simulink model "SERIALMASTERUPDATED"  (R2022b)
settings: Solver=FixedStepAuto  StartTime=0.0  StopTime=10.0  FixedStep=1e-3  RelTol=1e-3  EnableMultiTasking=on
undefined symbols (not defined in the file): D0, D1, D10, D11, D12, D13, D2, D3, D4, D5, D6, D7, D8, D9, PTA0, PTA1, PTA2, PTB23, PTB9, PTC16, PTC17, PTC2, PTC3, PTC4, PTD0, PTD1, PTD2, PTD3
libraries: frdmk64flib x18, etargetslib x12
settings Model: ExtModeTrigDuration=5  Creator=Riley  LastModifiedBy=Tiren
settings OptimizationCC: EnhancedBackFolding=on  PassReuseOutputArgsAs=Individual arguments  ZeroExternalMemoryAtStartup=off  ZeroInternalMemoryAtStartup=off  MaxStackSize=64  OptimizeBlockOrder=speed  DifferentSizesBufferReuse=on  OptimizationCustomize=off  EfficientTunableParamExpr=on
settings DebuggingCC: ParameterTunabilityLossMsg=error  UnconnectedInputMsg=warning  UnconnectedOutputMsg=warning  UnconnectedLineMsg=warning
settings HardwareCC: ProdBitPerPointer=32  ProdBitPerSizeT=32  ProdBitPerPtrDiffT=32  ProdLargestAtomicInteger=Long  ProdLargestAtomicFloat=Double  ProdWordSize=32  ProdHWDeviceType=ARM Compatible->ARM Cortex
settings ModelReferenceCC: EnableRefExpFcnMdlSchedulingChecks=on
settings SFSimCC: MATLABDynamicMemAlloc=off
settings RTWCC: Description=Embedded Coder  SystemTargetFile=ert.tlc  HardwareBoard=NXP FRDM-K64F  TLCOptions="-aInlineSetEventsForThisBaseRateFcn=TLC_FALSE -aSuppressMultiTaskScheduler=TLC_FALSE  -aRateBasedStepFcn=0"  TemplateMakefile=ert_default_tmf  Toolchain=GNU Tools for ARM Embedded Processors  DLArmComputeVersion=19.05
settings CodeAppCC: ForceParamTrailComments=on  IgnoreCustomStorageClasses=off  OperatorAnnotations=on  SimulinkDataObjDesc=on  SFDataObjDesc=on  InsertBlockDesc=on
settings ERTTargetCC: ExtModeTransport=4  ExtModeMexFile=sendToCommService

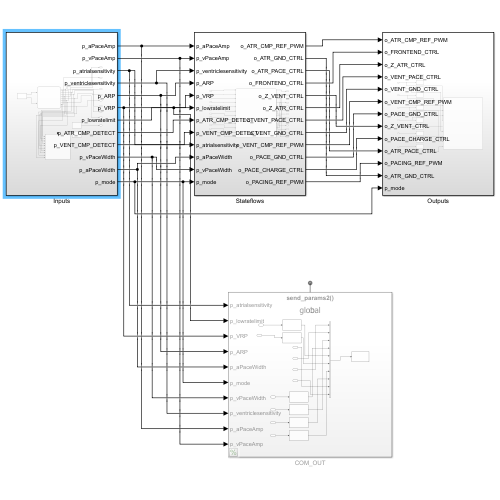
[thumbnail: Simulink's stored preview of the top-level diagram]
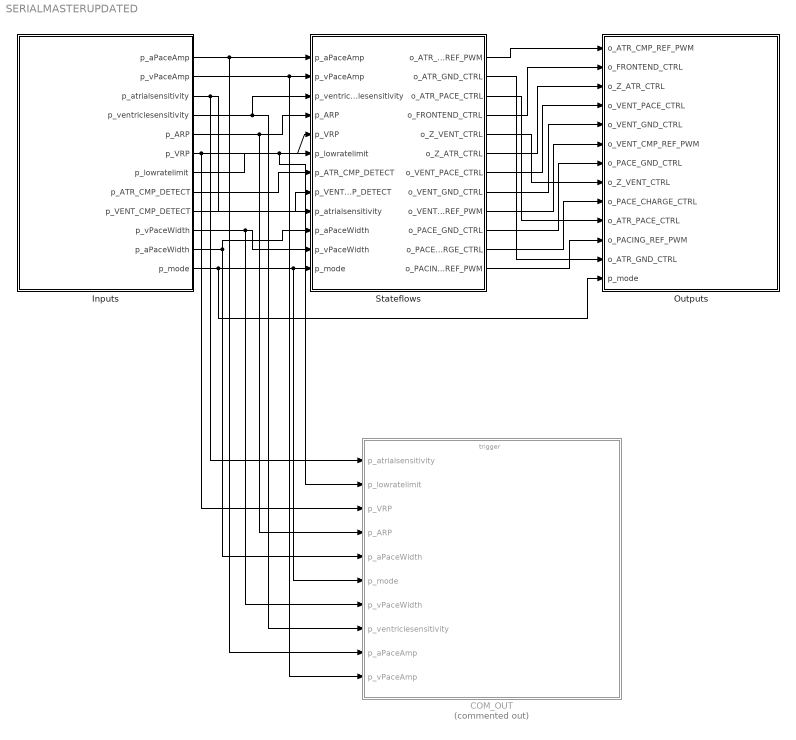
== system SERIALMASTERUPDATED ==
  COM_OUT : Subsystem  Commented=on  TreatAsAtomicUnit=on
  Inputs : Subsystem
  Outputs : Subsystem
  Stateflows : Subsystem
  wires:
  Inputs/1(p_aPaceAmp) -> COM_OUT/9(p_aPaceAmp), Stateflows/1(p_aPaceAmp)
  Inputs/2(p_vPaceAmp) -> COM_OUT/10(p_vPaceAmp), Stateflows/2(p_vPaceAmp)
  Inputs/3(p_atrialsensitivity) -> COM_OUT/1(p_atrialsensitivity), Stateflows/9(p_atrialsensitivity)
  Inputs/4(p_ventriclesensitivity) -> COM_OUT/8(p_ventriclesensitivity), Stateflows/3(p_ventriclesensitivity)
  Inputs/5(p_ARP) -> COM_OUT/4(p_ARP), Stateflows/4(p_ARP)
  Inputs/6(p_VRP) -> COM_OUT/3(p_VRP), Stateflows/5(p_VRP)
  Inputs/7(p_lowratelimit) -> COM_OUT/2(p_lowratelimit), Stateflows/6(p_lowratelimit)
  Inputs/8(p_ATR_CMP_DETECT) -> Stateflows/7(p_ATR_CMP_DETECT)
  Inputs/9(p_VENT_CMP_DETECT) -> Stateflows/8(p_VENT_CMP_DETECT)
  Inputs/10(p_vPaceWidth) -> COM_OUT/7(p_vPaceWidth), Stateflows/11(p_vPaceWidth)
  Inputs/11(p_aPaceWidth) -> COM_OUT/5(p_aPaceWidth), Stateflows/10(p_aPaceWidth)
  Inputs/12(p_mode) -> Outputs/13(p_mode), COM_OUT/6(p_mode), Stateflows/12(p_mode)
  Stateflows/1(o_ATR_CMP_REF_PWM) -> Outputs/1(o_ATR_CMP_REF_PWM)
  Stateflows/2(o_ATR_GND_CTRL) -> Outputs/12(o_ATR_GND_CTRL)
  Stateflows/3(o_ATR_PACE_CTRL) -> Outputs/10(o_ATR_PACE_CTRL)
  Stateflows/4(o_FRONTEND_CTRL) -> Outputs/2(o_FRONTEND_CTRL)
  Stateflows/5(o_Z_VENT_CTRL) -> Outputs/8(o_Z_VENT_CTRL)
  Stateflows/6(o_Z_ATR_CTRL) -> Outputs/3(o_Z_ATR_CTRL)
  Stateflows/7(o_VENT_PACE_CTRL) -> Outputs/4(o_VENT_PACE_CTRL)
  Stateflows/8(o_VENT_GND_CTRL) -> Outputs/5(o_VENT_GND_CTRL)
  Stateflows/9(o_VENT_CMP_REF_PWM) -> Outputs/6(o_VENT_CMP_REF_PWM)
  Stateflows/10(o_PACE_GND_CTRL) -> Outputs/7(o_PACE_GND_CTRL)
  Stateflows/11(o_PACE_CHARGE_CTRL) -> Outputs/9(o_PACE_CHARGE_CTRL)
  Stateflows/12(o_PACING_REF_PWM) -> Outputs/11(o_PACING_REF_PWM)

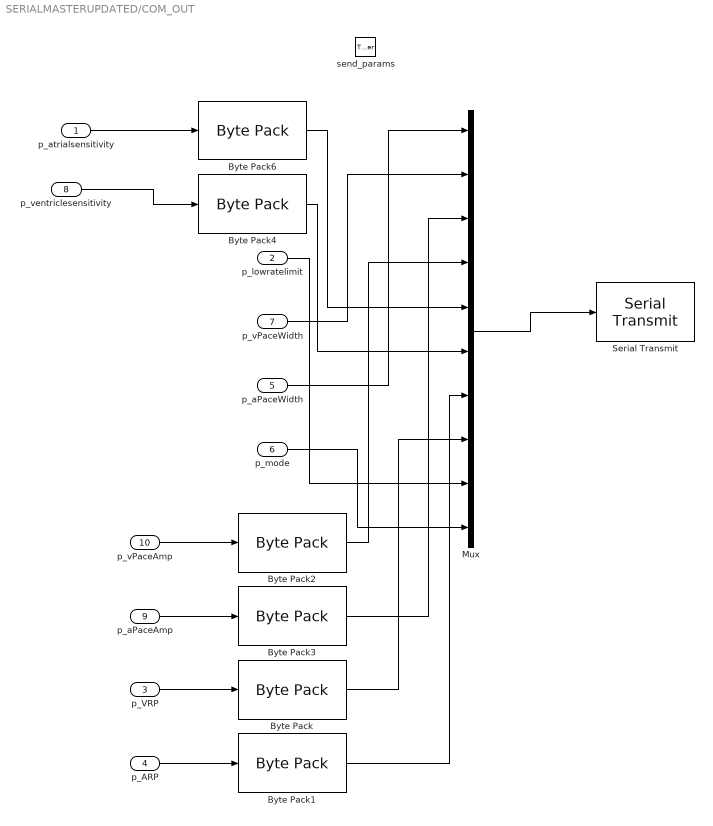
== system SERIALMASTERUPDATED/COM_OUT ==
  p_atrialsensitivity : Inport  OutDataTypeStr=single
  p_lowratelimit : Inport  Port=2  OutDataTypeStr=uint8
  p_VRP : Inport  Port=3  OutDataTypeStr=uint16
  p_ARP : Inport  Port=4  OutDataTypeStr=uint16
  p_aPaceWidth : Inport  Port=5  OutDataTypeStr=uint8
  p_mode : Inport  Port=6  OutDataTypeStr=uint8
  p_vPaceWidth : Inport  Port=7  OutDataTypeStr=uint8
  p_ventriclesensitivity : Inport  Port=8  OutDataTypeStr=single
  p_aPaceAmp : Inport  Port=9  OutDataTypeStr=single
  p_vPaceAmp : Inport  Port=10  OutDataTypeStr=single
  send_params : TriggerPort  TriggerType=function-call  IsSimulinkFunction=on  FunctionName=send_params2  VariantControl=(inherit)
  Byte Pack : etargetslib/Byte Pack  datatypes={'uint16'}  byteAlign=1
  Byte Pack1 : etargetslib/Byte Pack  datatypes={'uint16'}  byteAlign=1
  Byte Pack{2..4,6} (4 alike) : etargetslib/Byte Pack  datatypes={'single'}  byteAlign=1
  Mux : Mux  Inputs=10
  Serial Transmit : frdmk64flib/Serial Transmit  SCIModule=0  Baudrate=uint32(9600)  Parity=None  StopBits=1  HardwareFlowControl=None  ByteOrder=LittleEndian  BlockingMode=on  OutputStatus=off
  wires:
  Mux/1 -> Serial Transmit/1
  p_VRP/1 -> Byte Pack/1
  p_ARP/1 -> Byte Pack1/1
  p_vPaceAmp/1 -> Byte Pack2/1
  p_aPaceAmp/1 -> Byte Pack3/1
  p_atrialsensitivity/1 -> Byte Pack6/1
  p_ventriclesensitivity/1 -> Byte Pack4/1
  p_aPaceWidth/1 -> Mux/1
  p_vPaceWidth/1 -> Mux/2
  Byte Pack3/1 -> Mux/3
  Byte Pack2/1 -> Mux/4
  Byte Pack6/1 -> Mux/5
  Byte Pack4/1 -> Mux/6
  Byte Pack1/1 -> Mux/7
  Byte Pack/1 -> Mux/8
  p_lowratelimit/1 -> Mux/9
  p_mode/1 -> Mux/10

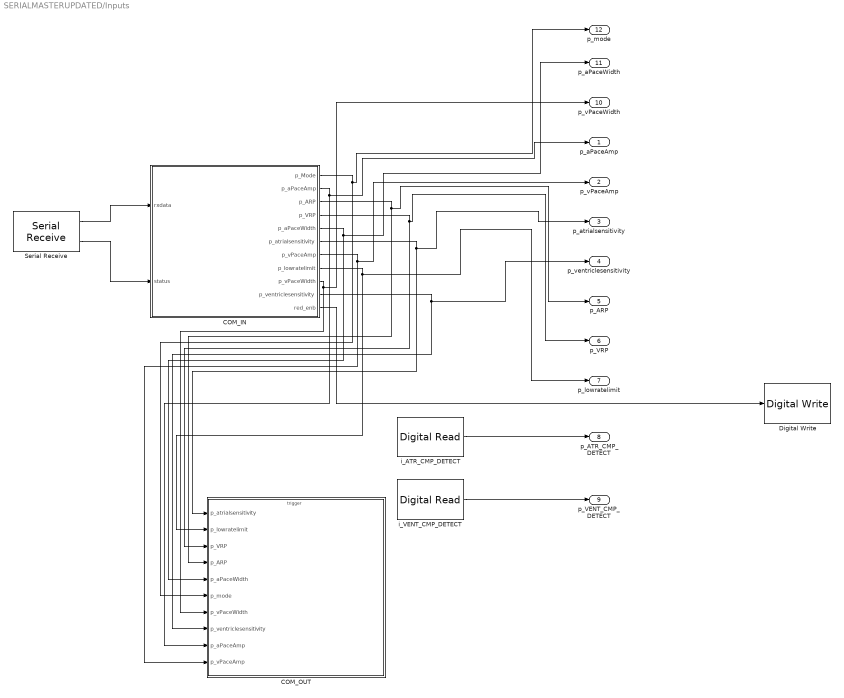
== system SERIALMASTERUPDATED/Inputs ==
  COM_IN : Stateflow chart  TreatAsAtomicUnit=on
  COM_OUT : Subsystem  TreatAsAtomicUnit=on
  Digital Write : frdmk64flib/Digital Write  Whichpin=RED_LED
  Serial Receive : frdmk64flib/Serial Receive  SCIModule=0  Baudrate=uint32(9600)  Parity=None  StopBits=1  HardwareFlowControl=None  ByteOrder=LittleEndian  DataType=uint8  DataLength=26  BlockingMode=off  OutputStatus=on  SampleTime=0.1
  i_ATR_CMP_DETECT : frdmk64flib/Digital Read  Whichpin=PTC16 (D0)  SampleTime=-1
  i_VENT_CMP_DETECT : frdmk64flib/Digital Read  Whichpin=PTC17 (D1)  SampleTime=-1
  p_aPaceAmp : Outport  OutDataTypeStr=single  Unit=mV
  p_vPaceAmp : Outport  Port=2  OutDataTypeStr=single  Unit=mV
  p_atrialsensitivity : Outport  Port=3  OutDataTypeStr=single  Unit=mV
  p_ventriclesensitivity : Outport  Port=4  OutDataTypeStr=single  Unit=mV
  p_ARP : Outport  Port=5  OutDataTypeStr=uint16  Unit=msec
  p_VRP : Outport  Port=6  OutDataTypeStr=uint16  Unit=msec
  p_lowratelimit : Outport  Port=7  OutDataTypeStr=uint8  Unit=msec
  p_ATR_CMP_DETECT : Outport  Port=8  OutDataTypeStr=boolean
  p_VENT_CMP_DETECT : Outport  Port=9  OutDataTypeStr=boolean
  p_vPaceWidth : Outport  Port=10  OutDataTypeStr=uint8  Unit=msec
  p_aPaceWidth : Outport  Port=11  OutDataTypeStr=uint8  Unit=msec
  p_mode : Outport  Port=12  OutDataTypeStr=uint8
  wires:
  i_ATR_CMP_DETECT/1 -> p_ATR_CMP_DETECT/1
  i_VENT_CMP_DETECT/1 -> p_VENT_CMP_DETECT/1
  Serial Receive/1 -> COM_IN/1(rxdata)
  Serial Receive/2 -> COM_IN/2(status)
  COM_IN/1(p_Mode) -> COM_OUT/6(p_mode), p_mode/1
  COM_IN/3(p_ARP) -> COM_OUT/4(p_ARP), p_ARP/1
  COM_IN/4(p_VRP) -> COM_OUT/3(p_VRP), p_VRP/1
  COM_IN/2(p_aPaceAmp) -> COM_OUT/9(p_aPaceAmp), p_aPaceAmp/1
  COM_IN/5(p_aPaceWidth) -> COM_OUT/5(p_aPaceWidth), p_aPaceWidth/1
  COM_IN/6(p_atrialsensitivity) -> COM_OUT/1(p_atrialsensitivity), p_atrialsensitivity/1
  COM_IN/8(p_lowratelimit) -> COM_OUT/2(p_lowratelimit), p_lowratelimit/1
  COM_IN/10(p_ventriclesensitivity) -> COM_OUT/8(p_ventriclesensitivity), p_ventriclesensitivity/1
  COM_IN/9(p_vPaceWidth) -> COM_OUT/7(p_vPaceWidth), p_vPaceWidth/1
  COM_IN/7(p_vPaceAmp) -> p_vPaceAmp/1, COM_OUT/10(p_vPaceAmp)
  COM_IN/11(red_enb) -> Digital Write/1

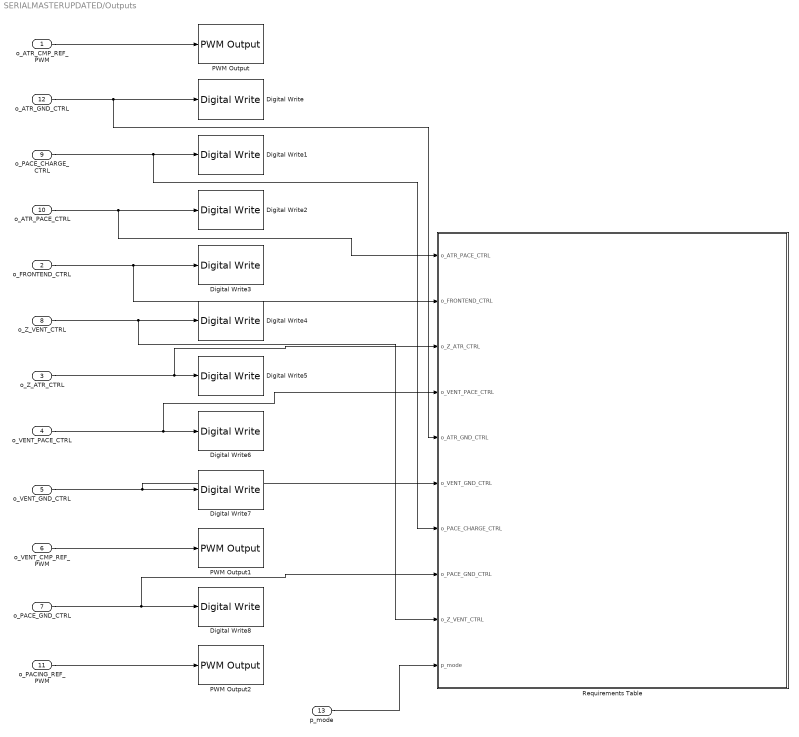
== system SERIALMASTERUPDATED/Outputs ==
  o_ATR_CMP_REF_PWM : Inport  OutDataTypeStr=single
  o_FRONTEND_CTRL : Inport  Port=2  OutDataTypeStr=boolean
  o_Z_ATR_CTRL : Inport  Port=3  OutDataTypeStr=boolean
  o_VENT_PACE_CTRL : Inport  Port=4  OutDataTypeStr=boolean
  o_VENT_GND_CTRL : Inport  Port=5  OutDataTypeStr=boolean
  o_VENT_CMP_REF_PWM : Inport  Port=6  OutDataTypeStr=single
  o_PACE_GND_CTRL : Inport  Port=7  OutDataTypeStr=boolean
  o_Z_VENT_CTRL : Inport  Port=8  OutDataTypeStr=boolean
  o_PACE_CHARGE_CTRL : Inport  Port=9  OutDataTypeStr=boolean
  o_ATR_PACE_CTRL : Inport  Port=10  OutDataTypeStr=boolean
  o_PACING_REF_PWM : Inport  Port=11  OutDataTypeStr=single
  o_ATR_GND_CTRL : Inport  Port=12  OutDataTypeStr=boolean
  p_mode : Inport  Port=13  OutDataTypeStr=uint8
  Digital Write : frdmk64flib/Digital Write  Whichpin=PTD2 (D11)
  Digital Write1 : frdmk64flib/Digital Write  Whichpin=PTB9 (D2)
  Digital Write2 : frdmk64flib/Digital Write  Whichpin=PTA0 (D8)
  Digital Write3 : frdmk64flib/Digital Write  Whichpin=PTD1 (D13)
  Digital Write4 : frdmk64flib/Digital Write  Whichpin=PTC3 (D7)
  Digital Write5 : frdmk64flib/Digital Write  Whichpin=PTB23 (D4)
  Digital Write6 : frdmk64flib/Digital Write  Whichpin=PTC4 (D9)
  Digital Write7 : frdmk64flib/Digital Write  Whichpin=PTD3 (D12)
  Digital Write8 : frdmk64flib/Digital Write  Whichpin=PTD0 (D10)
  PWM Output : frdmk64flib/PWM Output  Whichpin=PTC2 (D6)  InitialFrequency=2000  InitialDutyCycle=0
  PWM Output1 : frdmk64flib/PWM Output  Whichpin=PTA1 (D3)  InitialFrequency=2000  InitialDutyCycle=0
  PWM Output2 : frdmk64flib/PWM Output  Whichpin=PTA2 (D5)  InitialFrequency=2000  InitialDutyCycle=0
  Requirements Table : Requirements Table  TreatAsAtomicUnit=on
  wires:
  o_ATR_CMP_REF_PWM/1 -> PWM Output/1
  o_ATR_GND_CTRL/1 -> Requirements Table/5(o_ATR_GND_CTRL), Digital Write/1
  o_PACE_CHARGE_CTRL/1 -> Requirements Table/7(o_PACE_CHARGE_CTRL), Digital Write1/1
  o_ATR_PACE_CTRL/1 -> Requirements Table/1(o_ATR_PACE_CTRL), Digital Write2/1
  o_FRONTEND_CTRL/1 -> Requirements Table/2(o_FRONTEND_CTRL), Digital Write3/1
  o_Z_VENT_CTRL/1 -> Requirements Table/9(o_Z_VENT_CTRL), Digital Write4/1
  o_Z_ATR_CTRL/1 -> Requirements Table/3(o_Z_ATR_CTRL), Digital Write5/1
  o_VENT_PACE_CTRL/1 -> Requirements Table/4(o_VENT_PACE_CTRL), Digital Write6/1
  o_VENT_GND_CTRL/1 -> Requirements Table/6(o_VENT_GND_CTRL), Digital Write7/1
  o_VENT_CMP_REF_PWM/1 -> PWM Output1/1
  o_PACE_GND_CTRL/1 -> Requirements Table/8(o_PACE_GND_CTRL), Digital Write8/1
  o_PACING_REF_PWM/1 -> PWM Output2/1
  p_mode/1 -> Requirements Table/10(p_mode)

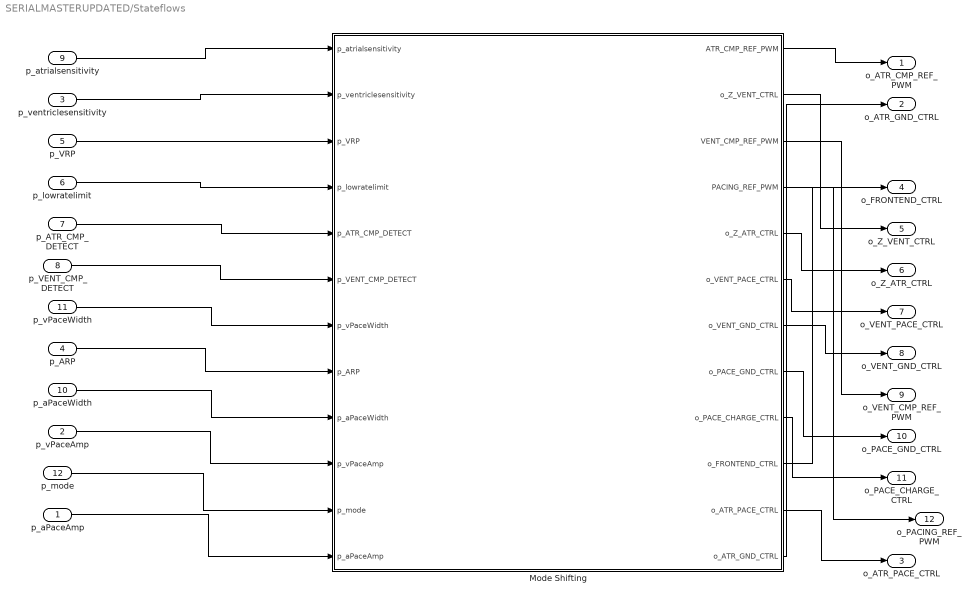
== system SERIALMASTERUPDATED/Stateflows ==
  p_aPaceAmp : Inport  OutDataTypeStr=single
  p_vPaceAmp : Inport  Port=2  OutDataTypeStr=single
  p_ventriclesensitivity : Inport  Port=3  OutDataTypeStr=single
  p_ARP : Inport  Port=4  OutDataTypeStr=uint16
  p_VRP : Inport  Port=5  OutDataTypeStr=uint16
  p_lowratelimit : Inport  Port=6  OutDataTypeStr=uint8
  p_ATR_CMP_DETECT : Inport  Port=7  OutDataTypeStr=boolean
  p_VENT_CMP_DETECT : Inport  Port=8  OutDataTypeStr=boolean
  p_atrialsensitivity : Inport  Port=9  OutDataTypeStr=single
  p_aPaceWidth : Inport  Port=10  OutDataTypeStr=uint8
  p_vPaceWidth : Inport  Port=11  OutDataTypeStr=uint8
  p_mode : Inport  Port=12  OutDataTypeStr=uint8
  Mode Shifting : Stateflow chart  TreatAsAtomicUnit=on
  o_ATR_CMP_REF_PWM : Outport  OutDataTypeStr=single
  o_ATR_GND_CTRL : Outport  Port=2  OutDataTypeStr=boolean
  o_ATR_PACE_CTRL : Outport  Port=3  OutDataTypeStr=boolean
  o_FRONTEND_CTRL : Outport  Port=4  OutDataTypeStr=boolean
  o_Z_VENT_CTRL : Outport  Port=5  OutDataTypeStr=boolean
  o_Z_ATR_CTRL : Outport  Port=6  OutDataTypeStr=boolean
  o_VENT_PACE_CTRL : Outport  Port=7  OutDataTypeStr=boolean
  o_VENT_GND_CTRL : Outport  Port=8  OutDataTypeStr=boolean
  o_VENT_CMP_REF_PWM : Outport  Port=9  OutDataTypeStr=single
  o_PACE_GND_CTRL : Outport  Port=10  OutDataTypeStr=boolean
  o_PACE_CHARGE_CTRL : Outport  Port=11  OutDataTypeStr=boolean
  o_PACING_REF_PWM : Outport  Port=12  OutDataTypeStr=single
  wires:
  p_aPaceAmp/1 -> Mode Shifting/12(p_aPaceAmp)
  p_vPaceAmp/1 -> Mode Shifting/10(p_vPaceAmp)
  p_atrialsensitivity/1 -> Mode Shifting/1(p_atrialsensitivity)
  p_ventriclesensitivity/1 -> Mode Shifting/2(p_ventriclesensitivity)
  p_ARP/1 -> Mode Shifting/8(p_ARP)
  p_VRP/1 -> Mode Shifting/3(p_VRP)
  p_lowratelimit/1 -> Mode Shifting/4(p_lowratelimit)
  p_ATR_CMP_DETECT/1 -> Mode Shifting/5(p_ATR_CMP_DETECT)
  p_VENT_CMP_DETECT/1 -> Mode Shifting/6(p_VENT_CMP_DETECT)
  p_vPaceWidth/1 -> Mode Shifting/7(p_vPaceWidth)
  p_aPaceWidth/1 -> Mode Shifting/9(p_aPaceWidth)
  p_mode/1 -> Mode Shifting/11(p_mode)
  Mode Shifting/1(ATR_CMP_REF_PWM) -> o_ATR_CMP_REF_PWM/1
  Mode Shifting/2(o_Z_VENT_CTRL) -> o_Z_VENT_CTRL/1
  Mode Shifting/3(VENT_CMP_REF_PWM) -> o_VENT_CMP_REF_PWM/1
  Mode Shifting/4(PACING_REF_PWM) -> o_PACING_REF_PWM/1
  Mode Shifting/5(o_Z_ATR_CTRL) -> o_Z_ATR_CTRL/1
  Mode Shifting/6(o_VENT_PACE_CTRL) -> o_VENT_PACE_CTRL/1
  Mode Shifting/7(o_VENT_GND_CTRL) -> o_VENT_GND_CTRL/1
  Mode Shifting/8(o_PACE_GND_CTRL) -> o_PACE_GND_CTRL/1
  Mode Shifting/9(o_PACE_CHARGE_CTRL) -> o_PACE_CHARGE_CTRL/1
  Mode Shifting/10(o_FRONTEND_CTRL) -> o_FRONTEND_CTRL/1
  Mode Shifting/11(o_ATR_PACE_CTRL) -> o_ATR_PACE_CTRL/1
  Mode Shifting/12(o_ATR_GND_CTRL) -> o_ATR_GND_CTRL/1

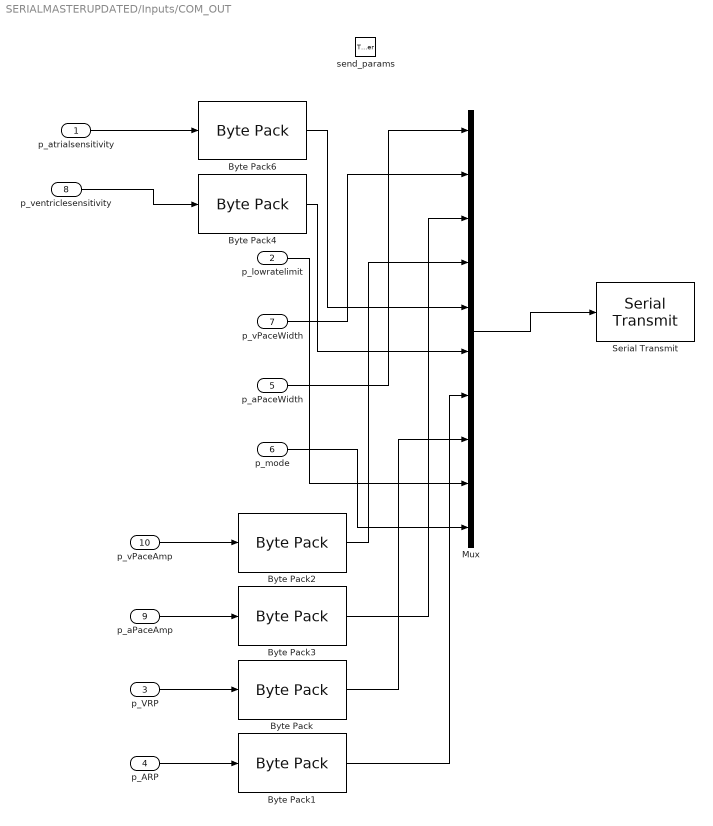
== system SERIALMASTERUPDATED/Inputs/COM_OUT ==
  p_atrialsensitivity : Inport  OutDataTypeStr=single
  p_lowratelimit : Inport  Port=2  OutDataTypeStr=uint8
  p_VRP : Inport  Port=3  OutDataTypeStr=uint16
  p_ARP : Inport  Port=4  OutDataTypeStr=uint16
  p_aPaceWidth : Inport  Port=5  OutDataTypeStr=uint8
  p_mode : Inport  Port=6  OutDataTypeStr=uint8
  p_vPaceWidth : Inport  Port=7  OutDataTypeStr=uint8
  p_ventriclesensitivity : Inport  Port=8  OutDataTypeStr=single
  p_aPaceAmp : Inport  Port=9  OutDataTypeStr=single
  p_vPaceAmp : Inport  Port=10  OutDataTypeStr=single
  send_params : TriggerPort  TriggerType=function-call  IsSimulinkFunction=on  FunctionName=send_params2  VariantControl=(inherit)
  Byte Pack : etargetslib/Byte Pack  datatypes={'uint16'}  byteAlign=1
  Byte Pack1 : etargetslib/Byte Pack  datatypes={'uint16'}  byteAlign=1
  Byte Pack{2..4,6} (4 alike) : etargetslib/Byte Pack  datatypes={'single'}  byteAlign=1
  Mux : Mux  Inputs=10
  Serial Transmit : frdmk64flib/Serial Transmit  SCIModule=0  Baudrate=uint32(9600)  Parity=None  StopBits=1  HardwareFlowControl=None  ByteOrder=LittleEndian  BlockingMode=on  OutputStatus=off
  wires:
  Mux/1 -> Serial Transmit/1
  p_VRP/1 -> Byte Pack/1
  p_ARP/1 -> Byte Pack1/1
  p_vPaceAmp/1 -> Byte Pack2/1
  p_aPaceAmp/1 -> Byte Pack3/1
  p_atrialsensitivity/1 -> Byte Pack6/1
  p_ventriclesensitivity/1 -> Byte Pack4/1
  p_aPaceWidth/1 -> Mux/1
  p_vPaceWidth/1 -> Mux/2
  Byte Pack3/1 -> Mux/3
  Byte Pack2/1 -> Mux/4
  Byte Pack6/1 -> Mux/5
  Byte Pack4/1 -> Mux/6
  Byte Pack1/1 -> Mux/7
  Byte Pack/1 -> Mux/8
  p_lowratelimit/1 -> Mux/9
  p_mode/1 -> Mux/10

== stateflow chart SERIALMASTERUPDATED/Inputs/COM_IN ==
  state SET_PARAMETERS
    entry:
    p_aPaceWidth = rxdata(3);
    p_vPaceWidth = rxdata(4);
    p_aPaceAmp = typecast(rxdata(5:8),'single');
    p_vPaceAmp = typecast(rxdata(9:12),'single');
    p_atrialsensitivity = typecast(rxdata(13:16),'single');
    p_ventriclesensitivity = typecast(rxdata(17:20),'single');
    p_ARP = typecast(rxdata(21:22),'uint16');
    p_VRP =typecast(rxdata(23:24),'uint16');
    p_lowratelimit = rxdata(25);
    p_Mode = rxdata(26);
    %red_enb = 1;
  state INITIAL
    %Set the initial values of parameters
    entry:
    p_aPaceWidth = 5;
    p_vPaceWidth = 1;
    p_aPaceAmp = 1;
    p_vPaceAmp = 1;
    p_atrialsensitivity = 1;
    p_ventriclesensitivity = 1;
    p_ARP = 1;
    p_VRP = 1;
    p_lowratelimit = 1;
    p_Mode =1;
    red_enb = 0;
  state STANDBY
    %wait for COM
  state ECHO_PARAMETERS
    entry:
    send_params2();
    red_enb = 1;
  SET_PARAMETERS -> STANDBY
  (default) -> INITIAL
  (junction 12) -> SET_PARAMETERS [order 2] : [rxdata(2)==55]
  (junction 9) -> STANDBY [order 2]
  INITIAL -> STANDBY
  STANDBY -> (junction 9) : [status == 0]
  (junction 9) -> (junction 12) [order 1] : [rxdata(1) == hex2dec('16')]
  (junction 12) -> ECHO_PARAMETERS [order 1] : [rxdata(2)==hex2dec('22')]
  ECHO_PARAMETERS -> STANDBY
  data: rxdata input uint8; status input uint8; p_Mode output uint8; p_aPaceAmp output single; p_ARP output uint16; p_VRP output uint16; p_aPaceWidth output uint8; p_atrialsensitivity output single; p_vPaceAmp output single; p_lowratelimit output uint8; p_vPaceWidth output uint8; p_ventriclesensitivity output single; red_enb output

== stateflow chart SERIALMASTERUPDATED/Stateflows/Mode Shifting ==
  state AOOPACING
    entry:
    %AV pacing
    o_PACE_CHARGE_CTRL= false;
    o_PACE_GND_CTRL = true;
    o_ATR_PACE_CTRL = true;
    o_ATR_GND_CTRL = false;
    o_VENT_GND_CTRL = false;
    o_VENT_PACE_CTRL =  false;
  state VOOPACING
    entry:
    %AV pacing
    o_PACE_CHARGE_CTRL= false;
    o_PACE_GND_CTRL = true;
    o_ATR_PACE_CTRL = false;
    o_ATR_GND_CTRL = false;
    o_VENT_GND_CTRL = false;
    o_VENT_PACE_CTRL =  true;
  state AAIPACINGHEART
    entry:
    %AV pacing
    o_PACE_CHARGE_CTRL= false;
    o_PACE_GND_CTRL = true;
    o_ATR_PACE_CTRL = true;
    o_ATR_GND_CTRL = false;
    o_VENT_GND_CTRL = false;
    o_VENT_PACE_CTRL =  false;
    %SENSING OFF
    o_FRONTEND_CTRL = false;
  state VVIPACINGHEART
    entry:
    %AV pacing
    o_PACE_CHARGE_CTRL= false;
    o_PACE_GND_CTRL = true;
    o_ATR_PACE_CTRL = false;
    o_ATR_GND_CTRL = false;
    o_VENT_GND_CTRL = false;
    o_VENT_PACE_CTRL =  true;
    %SENSING OFF
    o_FRONTEND_CTRL = false;
  state AAIDETECTION
    entry:
    %SENSING ON
    o_FRONTEND_CTRL = true;
  state VVIDETECTION
    entry:
    %SENSING ON
    o_FRONTEND_CTRL = true;
  state AOOCHARGINGDISCHARGING
    entry:
    %To charge C22
    o_ATR_PACE_CTRL = false;
    o_PACE_CHARGE_CTRL = true;
    %To discharge blocking capacitor
    entry:
    o_PACE_GND_CTRL = true;
    o_VENT_PACE_CTRL = false;
    o_ATR_PACE_CTRL = false;
    o_ATR_GND_CTRL = true;
  state VOOCHARGINGDISCHARGING
    entry:
    %To charge C22
    o_VENT_PACE_CTRL = false;
    o_PACE_CHARGE_CTRL = true;
    o_ATR_PACE_CTRL = false;
    %To discharge blocking capacitor
    entry:
    o_PACE_GND_CTRL = true;
    o_VENT_PACE_CTRL = false;
    o_ATR_PACE_CTRL = false;
    o_VENT_GND_CTRL = true;
  state AAICHARGINGDISCHARGING
    entry:
    %To charge C22
    o_ATR_PACE_CTRL = false;
    o_PACE_CHARGE_CTRL = true;
    %To discharge blocking capacitor
    entry:
    o_PACE_GND_CTRL = true;
    o_VENT_PACE_CTRL = false;
    o_ATR_PACE_CTRL = false;
    o_ATR_GND_CTRL = true;
  state VVICHARGINGDISCHARGING
    entry:
    %To charge C22
    o_VENT_PACE_CTRL = false;
    o_PACE_CHARGE_CTRL = true;
    o_ATR_PACE_CTRL = false;
    %To discharge blocking capacitor
    entry:
    o_PACE_GND_CTRL = true;
    o_VENT_PACE_CTRL = false;
    o_ATR_PACE_CTRL = false;
    o_VENT_GND_CTRL = true;
  state DEFAULTSTATE
    o_Z_ATR_CTRL = false;
    o_Z_VENT_CTRL = false;
    o_VENT_PACE_CTRL = false;
    o_ATR_PACE_CTRL = false;
    VPACING_REF_PWM = (p_vPaceAmp/5000)*100;
    APACING_REF_PWM = (p_aPaceAmp/5000)*100;
    o_FRONTEND_CTRL = false;
    ATR_CMP_REF_PWM = (p_atrialsensitivity/5000)*100;
    VENT_CMP_REF_PWM = (p_ventriclesensitivity/5000)*100;
    o_PACE_CHARGE_CTRL = false;
    o_ATR_GND_CTRL = false;
    o_VENT_GND_CTRL = false;
    o_PACE_GND_CTRL = false;
  VVIPACINGHEART -> VVICHARGINGDISCHARGING
  AAIPACINGHEART -> AAICHARGINGDISCHARGING : after(p_aPaceWidth,msec)
  AOOCHARGINGDISCHARGING -> AOOPACING : after(p_lowratelimit - p_aPaceWidth,msec)
  AOOPACING -> AOOCHARGINGDISCHARGING : after(p_aPaceWidth,msec)
  VOOCHARGINGDISCHARGING -> VOOPACING : after(p_lowratelimit - p_vPaceWidth,msec)
  VOOPACING -> VOOCHARGINGDISCHARGING : after(p_vPaceWidth,msec)
  AAIDETECTION -> AAIPACINGHEART [order 2] : after(p_lowratelimit-p_aPaceWidth-uint8(p_ARP),msec)
  VVIDETECTION -> VVIPACINGHEART [order 2] : after(p_lowratelimit-p_vPaceWidth-uint8(p_VRP),msec)
  VVIDETECTION -> VVICHARGINGDISCHARGING [order 1] : [p_VENT_CMP_DETECT == true]
  AAIDETECTION -> AAICHARGINGDISCHARGING [order 1] : [p_ATR_CMP_DETECT == true]
  AAICHARGINGDISCHARGING -> AAIDETECTION : after(p_ARP,msec)
  VVICHARGINGDISCHARGING -> VVIDETECTION : after(p_VRP,msec)
  DEFAULTSTATE -> AOOCHARGINGDISCHARGING [order 2] : [p_mode == 1]{PACING_REF_PWM = APACING_REF_PWM}
  DEFAULTSTATE -> VOOCHARGINGDISCHARGING [order 1] : [p_mode == 2 ]{PACING_REF_PWM = APACING_REF_PWM}
  DEFAULTSTATE -> AAICHARGINGDISCHARGING [order 3] : [p_mode == 3]{PACING_REF_PWM = VPACING_REF_PWM}
  DEFAULTSTATE -> VVICHARGINGDISCHARGING [order 4] : [p_mode == 4]{PACING_REF_PWM = VPACING_REF_PWM}
  (default) -> DEFAULTSTATE
  data: p_atrialsensitivity input single; p_ventriclesensitivity input single; p_VRP input uint16; p_lowratelimit input uint8; p_ATR_CMP_DETECT input boolean; p_VENT_CMP_DETECT input boolean; p_vPaceWidth input uint8; p_ARP input uint16; p_aPaceWidth input uint8; p_vPaceAmp input single; p_mode input uint8; p_aPaceAmp input single; ATR_CMP_REF_PWM output single; o_Z_VENT_CTRL output boolean; VENT_CMP_REF_PWM output single; PACING_REF_PWM output single; APACING_REF_PWM local single; VPACING_REF_PWM local single; o_Z_ATR_CTRL output boolean; o_VENT_PACE_CTRL output boolean; o_VENT_GND_CTRL output boolean; o_PACE_GND_CTRL output boolean; o_PACE_CHARGE_CTRL output boolean; o_FRONTEND_CTRL output boolean; o_ATR_PACE_CTRL output boolean; o_ATR_GND_CTRL output boolean

== stateflow chart SERIALMASTERUPDATED/Outputs/Requirements Table ==
  (default) -> (junction 1073742986)
  (junction 1073742986) -> (junction 1073742987) : {
      | % SF_REQ_REV_07
      | }
  (junction 1073742987) -> (junction 1073742989) : {
      | % HEADER_ASSIGNMENTS
      |
      | }
  (junction 1073742989) -> (junction 1073742991) : {
      | % START_A_4
      | }
  (junction 1073742991) -> (junction 1073742993) : {
      | }
  (junction 1073742993) -> (junction 1073742995)
  (junction 1073742995) -> (junction 1073742997) : {
      | }
  (junction 1073742997) -> (junction 1073742999) : {
      | % END_A_4
      | }
  (junction 1073742999) -> (junction 1073743001) : {
      | % START_R_1
      | }
  (junction 1073743001) -> (junction 1073743003) : {
      | }
  (junction 1073743003) -> (junction 1073743005)
  (junction 1073743005) -> (junction 1073743007) [order 1] : [(p_mode == 1||p_mode == 3) && (((o_PACE_GND_CTRL) == (1))) && (((o_PACE_CHARGE_CTRL) == (1)))]
  (junction 1073743005) -> (junction 1073743013) [order 2]
  (junction 1073743007) -> (junction 1073743009) : {
      | reqtable_postcondition((((o_ATR_GND_CTRL) == (1))) && (((o_ATR_PACE_CTRL) == (0))) && (((o_Z_VENT_CTRL) == (0))) && (((o_Z_ATR_CTRL) == (0))) && (((o_VENT_PACE_CTRL) == (0))) && (((o_VENT_GND_CTRL) == (0))), 'R:1');
      |
      |
      | }
  (junction 1073743009) -> (junction 1073743011) : {
      | }
  (junction 1073743011) -> (junction 1073743013)
  (junction 1073743013) -> (junction 1073743015)
  (junction 1073743015) -> (junction 1073743017) : {
      | % END_R_1
      | }
  (junction 1073743017) -> (junction 1073743019) : {
      | % START_R_7
      | }
  (junction 1073743019) -> (junction 1073743021) : {
      | }
  (junction 1073743021) -> (junction 1073743023)
  (junction 1073743023) -> (junction 1073743025) [order 1] : [(p_mode == 1||p_mode == 3) && (((o_PACE_GND_CTRL) == (1))) && (((o_PACE_CHARGE_CTRL) == (0)))]
  (junction 1073743023) -> (junction 1073743031) [order 2]
  (junction 1073743025) -> (junction 1073743027) : {
      | reqtable_postcondition((((o_ATR_GND_CTRL) == (0))) && (((o_ATR_PACE_CTRL) == (1))) && (((o_Z_VENT_CTRL) == (0))) && (((o_Z_ATR_CTRL) == (0))) && (((o_VENT_PACE_CTRL) == (0))) && (((o_VENT_GND_CTRL) == (0))), 'R:2');
      |
      |
      | }
  (junction 1073743027) -> (junction 1073743029) : {
      | }
  (junction 1073743029) -> (junction 1073743031)
  (junction 1073743031) -> (junction 1073743033)
  (junction 1073743033) -> (junction 1073743035) : {
      | % END_R_7
      | }
  (junction 1073743035) -> (junction 1073743037) : {
      | % START_R_10
      | }
  (junction 1073743037) -> (junction 1073743039) : {
      | }
  (junction 1073743039) -> (junction 1073743041)
  (junction 1073743041) -> (junction 1073743043) [order 1] : [(p_mode == 2||p_mode == 4) && (((o_PACE_GND_CTRL) == (1))) && (((o_PACE_CHARGE_CTRL) == (1)))]
  (junction 1073743041) -> (junction 1073743049) [order 2]
  (junction 1073743043) -> (junction 1073743045) : {
      | reqtable_postcondition((((o_ATR_GND_CTRL) == (0))) && (((o_ATR_PACE_CTRL) == (0))) && (((o_Z_VENT_CTRL) == (0))) && (((o_Z_ATR_CTRL) == (0))) && (((o_VENT_PACE_CTRL) == (0))) && (((o_VENT_GND_CTRL) == (1))), 'R:3');
      |
      |
      | }
  (junction 1073743045) -> (junction 1073743047) : {
      | }
  (junction 1073743047) -> (junction 1073743049)
  (junction 1073743049) -> (junction 1073743051)
  (junction 1073743051) -> (junction 1073743053) : {
      | % END_R_10
      | }
  (junction 1073743053) -> (junction 1073743055) : {
      | % START_R_13
      | }
  (junction 1073743055) -> (junction 1073743057) : {
      | }
  (junction 1073743057) -> (junction 1073743059)
  (junction 1073743059) -> (junction 1073743061) [order 1] : [(p_mode == 2|| p_mode == 4) && (((o_PACE_GND_CTRL) == (1))) && (((o_PACE_CHARGE_CTRL) == (0)))]
  (junction 1073743059) -> (junction 1073743067) [order 2]
  (junction 1073743061) -> (junction 1073743063) : {
      | reqtable_postcondition((((o_ATR_GND_CTRL) == (0))) && (((o_ATR_PACE_CTRL) == (0))) && (((o_Z_VENT_CTRL) == (0))) && (((o_Z_ATR_CTRL) == (0))) && (((o_VENT_PACE_CTRL) == (1))) && (((o_VENT_GND_CTRL) == (0))), 'R:4');
      |
      |
      | }
  (junction 1073743063) -> (junction 1073743065) : {
      | }
  (junction 1073743065) -> (junction 1073743067)
  (junction 1073743067) -> (junction 1073743069)
  (junction 1073743069) -> (junction 1073743071) : {
      | % END_R_13
      | }
  (junction 1073743071) -> (junction 1073743073) : {
      | % START_R_16
      | }
  (junction 1073743073) -> (junction 1073743075) : {
      | }
  (junction 1073743075) -> (junction 1073743077)
  (junction 1073743077) -> (junction 1073743079) [order 1] : [(((o_PACE_GND_CTRL) == (1))) && (((o_FRONTEND_CTRL) == (1)))]
  (junction 1073743077) -> (junction 1073743085) [order 2]
  (junction 1073743079) -> (junction 1073743081) : {
      | reqtable_postcondition((((o_ATR_PACE_CTRL) == (0))) && (((o_Z_VENT_CTRL) == (0))) && (((o_Z_ATR_CTRL) == (0))) && (((o_VENT_PACE_CTRL) == (0))), 'R:5');
      |
      |
      | }
  (junction 1073743081) -> (junction 1073743083) : {
      | }
  (junction 1073743083) -> (junction 1073743085)
  (junction 1073743085) -> (junction 1073743087)
  (junction 1073743087) -> (junction 1073743089) : {
      | % END_R_16
      | }
  (junction 1073743089) -> (junction 1073743110) : {
      | % START_R_25
      | }
  (junction 1073743110) -> (junction 1073743112) : {
      | }
  (junction 1073743112) -> (junction 1073743114)
  (junction 1073743114) -> (junction 1073743116) [order 1] : [(((o_PACE_GND_CTRL) == (0))) && (((o_PACE_CHARGE_CTRL) == (0))) && (((o_FRONTEND_CTRL) == (0)))]
  (junction 1073743114) -> (junction 1073743122) [order 2]
  (junction 1073743116) -> (junction 1073743118) : {
      | reqtable_postcondition((((o_ATR_GND_CTRL) == (0))) && (((o_ATR_PACE_CTRL) == (0))) && (((o_Z_VENT_CTRL) == (0))) && (((o_Z_ATR_CTRL) == (0))) && (((o_VENT_PACE_CTRL) == (0))) && (((o_VENT_GND_CTRL) == (0))), 'R:6');
      |
      |
      | }
  (junction 1073743118) -> (junction 1073743120) : {
      | }
  (junction 1073743120) -> (junction 1073743122)
  (junction 1073743122) -> (junction 1073743124)
  (junction 1073743124) -> (junction 1073743126) : {
      | % END_R_25
      | }
  data: o_ATR_PACE_CTRL input boolean; o_FRONTEND_CTRL input boolean; o_Z_ATR_CTRL input boolean; o_VENT_PACE_CTRL input boolean; o_ATR_GND_CTRL input boolean; o_VENT_GND_CTRL input boolean; o_PACE_CHARGE_CTRL input boolean; o_PACE_GND_CTRL input boolean; o_Z_VENT_CTRL input boolean; p_mode input uint8
